simulink model "DP_MotionRAO"  (Simulink 7.4)
settings: Solver=ode4  StartTime=0.0  StopTime=200  FixedStep=0.05  RelTol=1e-3
undefined symbols (not defined in the file): Hoerner, slcm, vessel
libraries: simulink_extras x6, marine_hydro x3, marine_gnc x3, simulink x1
settings Model: Creator=Thor  LastModifiedBy=Thor
settings OptimizationCC: InlineInvariantSignals=on  InitFltsAndDblsToZero=on
settings DebuggingCC: SaveWithParameterizedLinksMsg=none  SignalResolutionControl=TryResolveAllWithWarning  MultiTaskDSMMsg=warning  MultiTaskCondExecSysMsg=none  StrictBusMsg=None
settings RTWCC: IncludeERTFirstTime=on
settings GRTTargetCC: TargetFcnLib=ansi_tfl_tmw.mat

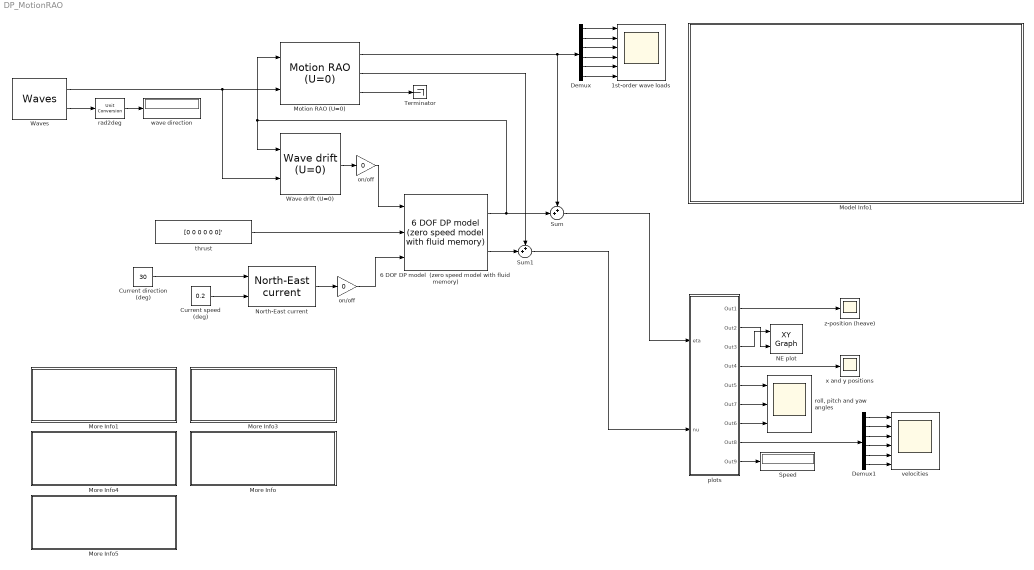
== system DP_MotionRAO ==
  "1st-order wave loads " : Scope  NumInputPorts=6
      settings: TimeRange=200  YMin=-2~-2~-2~-0.4~-0.1~-0.02  YMax=2~1~2~0.4~0.1~0.02
  6 DOF DP model  (zero speed model with fluid memory) : marine_hydro/Hydro Library/6 DOF DP model  (zero speed model with fluid memory)  SystemSampleTime=-1  ABC=vesselABC  rho=1025  Axc=106  Ayc=419  CX=1.0  CY_2D=Hoerner(vessel.main.B,vessel.main.T)  Bv=vessel.Bv
  Current direction (deg) : Constant  Value=30  OutDataType=sfix(16)  OutScaling=2^0
  Current speed (deg) : Constant  Value=0.2  OutDataType=sfix(16)  OutScaling=2^0
  Demux : Demux  Outputs=6
  Demux1 : Demux  Outputs=6
  Model Info1 : Subsystem  LoadFcn=slcm LoadBlock;  InitFcn=slcm('UpdateAllCMBlocksInThisModelInit')  mask(CMBlock){InitialSaveTempField=, InitialBlockCM=None, BlockCM=None, Frame=on, SaveTempField=, DisplayStringWithTags=|, MaskDisplayString=DP_MotionRAO.mdl template (Zero Speed DP Vessel Simulator using MOTION RAOs)\n\nSave this file to your working catalogue before you start editing\n\nVessel simulator for low-speed maneuvering and station-keeping in 6 DOF based on frequency-dependent\nhydrodynamic data. The wave loads and the fluid memory effects are computed using ShipX (VERES) or\nWAMIT that are postprocessed according to:\n\n>>vessel = veres2vessel ('input')        generates the vessel/hydrodynamic data structure <vessel> and *.mat \n>>vessel = wamit2vessel ('myship'')   generates the vessel/hydrodynamic data structure <vessel> and *.mat \n\n>>vesselABC = vessel2ss( vessel )     generates the fluid memory structure <vesselABC> and *ABC.mat\n\nThe data structures <vesselABC> and <vessel> must be in the workspace before starting the simulation\n\nDownload link: www.marinecontrol.org\n\nAuthor: Thor I. Fossen\n17-Sep-2009 10:25:38, HorizontalTextAlignment=Left, LeftAlignmentValue=0.02, SourceBlockDiagram=DP_MotionRAO, TagMaxNumber=20, CMTag1=, CMTag2=, CMTag3=, CMTag4=, CMTag5=, CMTag6=, CMTag7=, CMTag8=, CMTag9=, CMTag10=, CMTag11=, CMTag12=, CMTag13=, CMTag14=, CMTag15=, CMTag16=, CMTag17=, CMTag18=, CMTag19=, CMTag20=}
      mask DisplayStringWithTags=|
      | DP_MotionRAO.mdl template (Zero Speed DP Vessel Simulator using MOTION RAOs)\n
      | Save this file to your working catalogue before you start editing\n
      | Vessel simulator for low-speed maneuvering and station-keeping in 6 DOF based on frequency-dependent\nhydrodynamic data. The wave loads and the fluid memory effects are computed using ShipX (VERES) or\nWAMIT that are postprocessed according to:\n
      | >>vessel = veres2vessel ('input')        generates the vessel/hydrodynamic data structure <vessel> and *.mat
      | >>vessel = wamit2vessel ('myship'')   generates the vessel/hydrodynamic data structure <vessel> and *.mat
      |
      | >>vesselABC = vessel2ss( vessel )     generates the fluid memory structure <vesselABC> and *ABC.mat
      |
      | The data structures <vesselABC> and <vessel> must be in the workspace before starting the simulation
      |
      | Download link: www.marinecontrol.org
      |
      | Author: Thor I. Fossen
      | %<LastModificationDate>
      mask help: This block allows revision control information to be displayed within the model.
      settings: CopyFcn=slcm CopyBlock;  DeleteFcn=slcm Cancel;  PostSaveFcn=slcm('UpdateAllCMBlocksInThisModel')  NameChangeFcn=slcm Rename;  OpenFcn=slcm
      mask Display: text(str2num(LeftAlignmentValue), 0.5, MaskDisplayString, 'HorizontalAlignment', HorizontalTextAlignment)
  More Info : Subsystem
      settings: OpenFcn=load('supply'),load('supplyABC');disp('MSS supply vessel data set (L = 82.80 m) loaded')
      mask Display: disp('ShipX: Supply Vessel (L = 82.80 m)\n  Double-click to load the MSS data files:\n supply.mat\n supplyABC.mat')
  More Info1 : Subsystem
      settings: OpenFcn=load('tanker'),load('tankerABC');disp('MSS tanker data set (L = 246.0 m) loaded')
      mask Display: disp('WAMIT: Tanker (L = 246.0 m)\n  Double-click to load the MSS data files:\n tanker.mat\n tankerABC.mat')
  More Info3 : Subsystem
      settings: OpenFcn=load('s175'),load('s175ABC');disp('MSS S175 data set (L = 175.0 m) loaded')
      mask Display: disp('ShipX: S175 (L = 175.0 m)\n  Double-click to load the MSS data files:\n s175.mat\n s175ABC.mat')
  More Info4 : Subsystem
      settings: OpenFcn=load('fpso'),load('fpsoABC');disp('MSS FPSO data set (L = 200.0 m) loaded')
      mask Display: disp('WAMIT: FPSO (L = 200.0 m)\n  Double-click to load the MSS data files:\n fpso.mat\n fpsoABC.mat')
  More Info5 : Subsystem
      settings: OpenFcn=load('semisub'),load('semisubABC');disp('MSS semi-sub data set (L = 115.0 m) loaded')
      mask Display: disp('WAMIT: Semi-sub (L = 115.0 m)\n  Double-click to load the MSS data files:\n semisub.mat\n semisubABC.mat')
  Motion RAO (U=0) : marine_hydro/Hydro Library/Motion RAO (U=0)  SystemSampleTime=-1  RAO_Freq=vessel.motionRAO.w  RAO_Dir=vessel.headings  RAO_Vel=vessel.velocities  RAO_Amp=vessel.motionRAO.amp  RAO_Phase=vessel.motionRAO.phase  RAO_add_omega_0=on  RAO_add_omega_inf=on  RAO_yaw_quantization_flag=on  RAO_yaw_quant=5*pi/180  RAO_yaw_back=1.2*pi/180  RAO_speed_backlash_flag=on  RAO_speed_back=2  RAO_smoothing_flag=on
  NE plot : simulink/Sinks/XY Graph  SystemSampleTime=-1  xmin=-50  xmax=50  ymin=-50  ymax=50  st=-1
  North-East current : marine_gnc/Environment/Current/North-East current  SystemSampleTime=-1
  Speed : Display
  Sum : Sum  Inputs=++|  OutDataType=sfix(16)  OutScaling=2^0
  Sum1 : Sum  Inputs=++|  OutDataType=sfix(16)  OutScaling=2^0
  Terminator : Terminator
  Wave drift (U=0) : marine_hydro/Hydro Library/Wave drift (U=0)  SystemSampleTime=-1
  Waves : marine_gnc/Environment/Waves/Waves  SystemSampleTime=-1  spectrum_type=ITTC  disp_flag=off  plot_spectrum=off  plot_realization=off  hs=5  omega_peak=-1  psi_mean=30/(180/pi)  gamma=-1  spread=2  depth=inf  nfreq=20  ndir=10  energylim=0.005  freq_cutoff=3  dir_cutoff=0  rand_seed=0  rand_freq=on  rand_dir=on  Zeta_a=0  Omega=0  Phase=0  Wavenum=0  Psi=0
  on/off : Gain  Gain=0  ParameterDataType=sfix(16)  ParameterScaling=2^0  OutDataType=sfix(16)  OutScaling=2^0
  "on/off " : Gain  Gain=0  ParameterDataType=sfix(16)  ParameterScaling=2^0  OutDataType=sfix(16)  OutScaling=2^0
  plots : Subsystem
      mask Display: disp('time-series')
  rad2deg : marine_gnc/Utilities/Math Operations/Unit Conversion  SystemSampleTime=-1  in=rad2deg
  "roll, pitch and yaw angles" : Scope  NumInputPorts=3
      settings: TimeRange=200  YMin=-2~-4~-5  YMax=4~4~10
  thrust : Constant  Value=[0 0 0 0 0 0]'  OutDataType=sfix(16)  OutScaling=2^0
  velocities : Scope  NumInputPorts=6
      settings: TimeRange=200  YMin=-0.5~-0.4~-0.5~-5~-2.5~-1  YMax=0.6~0.5~0.5~5~2.5~1.25  SaveName=ScopeData4
  wave direction : Display
  x and y positions : Scope
      settings: TimeRange=200  YMin=-3  YMax=3  SaveName=ScopeData2
  z-position (heave) : Scope
      settings: TimeRange=200  YMin=-1  YMax=1  SaveName=ScopeData3
  wires:
  thrust/1 -> 6 DOF DP model  (zero speed model with fluid memory)/2
  6 DOF DP model  (zero speed model with fluid memory)/1 -> Sum/2, Motion RAO (U=0)/1, Wave drift (U=0)/1
  Demux/1 -> "1st-order wave loads "/1
  Demux/2 -> "1st-order wave loads "/2
  Demux/3 -> "1st-order wave loads "/3
  Demux/4 -> "1st-order wave loads "/4
  Demux/5 -> "1st-order wave loads "/5
  Demux/6 -> "1st-order wave loads "/6
  Waves/1 -> Motion RAO (U=0)/2, Wave drift (U=0)/2
  Waves/2 -> rad2deg/1
  rad2deg/1 -> wave direction/1
  Motion RAO (U=0)/1 -> Demux/1, Sum/1
  6 DOF DP model  (zero speed model with fluid memory)/2 -> Sum1/2
  Motion RAO (U=0)/2 -> Sum1/1
  Motion RAO (U=0)/3 -> Terminator/1
  North-East current/1 -> "on/off "/1
  "on/off "/1 -> 6 DOF DP model  (zero speed model with fluid memory)/3
  Current speed (deg)/1 -> North-East current/2
  Current direction (deg)/1 -> North-East current/1
  plots/3(Out3) -> NE plot/1
  plots/2(Out2) -> NE plot/2
  plots/4(Out4) -> x and y positions/1
  plots/5(Out5) -> "roll, pitch and yaw angles"/1
  plots/6(Out7) -> "roll, pitch and yaw angles"/2
  plots/7(Out6) -> "roll, pitch and yaw angles"/3
  plots/1(Out1) -> z-position (heave)/1
  Demux1/1 -> velocities/1
  Demux1/2 -> velocities/2
  Demux1/3 -> velocities/3
  Demux1/4 -> velocities/4
  Demux1/5 -> velocities/5
  Demux1/6 -> velocities/6
  Sum1/1 -> plots/2(nu)
  plots/8(Out8) -> Demux1/1
  plots/9(Out9) -> Speed/1
  Sum/1 -> plots/1(eta)
  on/off/1 -> 6 DOF DP model  (zero speed model with fluid memory)/1
  Wave drift (U=0)/1 -> on/off/1

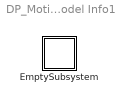
== system DP_MotionRAO/Model Info1 ==
  EmptySubsystem : Subsystem

== system DP_MotionRAO/More Info ==

== system DP_MotionRAO/More Info1 ==

== system DP_MotionRAO/More Info3 ==

== system DP_MotionRAO/More Info4 ==

== system DP_MotionRAO/More Info5 ==

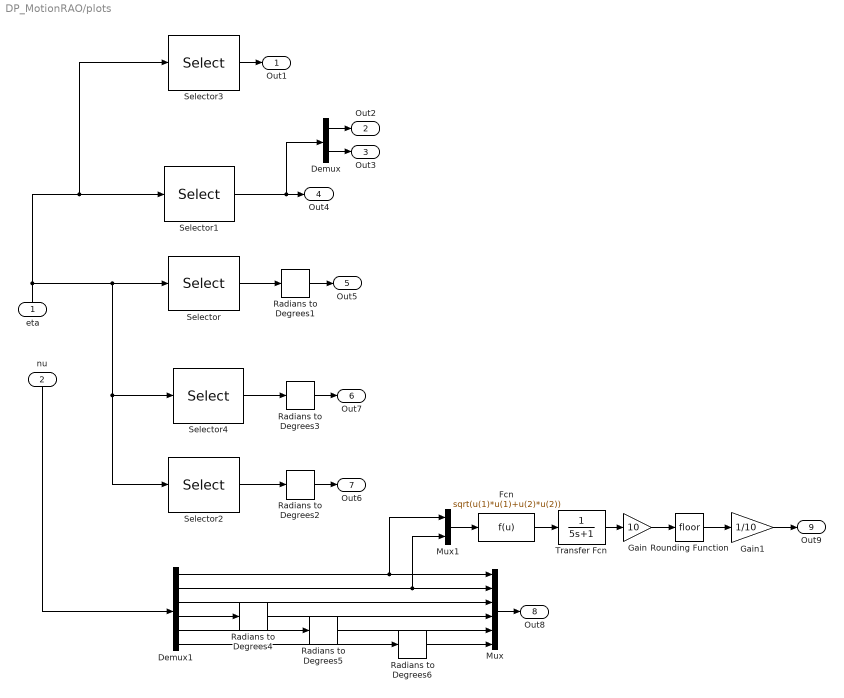
== system DP_MotionRAO/plots ==
  eta : Inport  OutDataType=sfix(16)  OutScaling=2^0
  nu : Inport  Port=2  OutDataType=sfix(16)  OutScaling=2^0
  Demux : Demux  Outputs=2
  Demux1 : Demux  Outputs=6
  Fcn : Fcn  Expr=sqrt(u(1)*u(1)+u(2)*u(2))
  Gain : Gain  Gain=10  ParameterDataType=sfix(16)  ParameterScaling=2^0  OutDataType=sfix(16)  OutScaling=2^0
  Gain1 : Gain  Gain=1/10  ParameterDataType=sfix(16)  ParameterScaling=2^0  OutDataType=sfix(16)  OutScaling=2^0
  Mux : Mux  Inputs=6
  Mux1 : Mux  Inputs=2
  Radians to Degrees{1..6} (6 alike) : simulink_extras/Transformations/Radians to Degrees  SystemSampleTime=-1
  Rounding Function : Rounding
  Selector : Selector  InputPortWidth=6  IndexOptions=Index vector (dialog)  Indices=[4 ]  OutputSizes=1
  Selector1 : Selector  InputPortWidth=6  IndexOptions=Index vector (dialog)  Indices=[1 2]  OutputSizes=1
  Selector2 : Selector  InputPortWidth=6  IndexOptions=Index vector (dialog)  Indices=[6]  OutputSizes=1
  Selector3 : Selector  InputPortWidth=6  IndexOptions=Index vector (dialog)  Indices=[3]  OutputSizes=1
  Selector4 : Selector  InputPortWidth=6  IndexOptions=Index vector (dialog)  Indices=[5]  OutputSizes=1
  Transfer Fcn : TransferFcn  Denominator=[5 1]
  Out1 : Outport  OutDataType=sfix(16)  OutScaling=2^0
  Out2 : Outport  Port=2  OutDataType=sfix(16)  OutScaling=2^0
  Out3 : Outport  Port=3  OutDataType=sfix(16)  OutScaling=2^0
  Out4 : Outport  Port=4  OutDataType=sfix(16)  OutScaling=2^0
  Out5 : Outport  Port=5  OutDataType=sfix(16)  OutScaling=2^0
  Out7 : Outport  Port=6  OutDataType=sfix(16)  OutScaling=2^0
  Out6 : Outport  Port=7  OutDataType=sfix(16)  OutScaling=2^0
  Out8 : Outport  Port=8  OutDataType=sfix(16)  OutScaling=2^0
  Out9 : Outport  Port=9  OutDataType=sfix(16)  OutScaling=2^0
  wires:
  eta/1 -> Selector3/1, Selector1/1, Selector/1, Selector2/1, Selector4/1
  Selector/1 -> Radians to Degrees1/1
  Selector1/1 -> Demux/1, Out4/1
  Selector2/1 -> Radians to Degrees2/1
  Selector3/1 -> Out1/1
  Demux/1 -> Out2/1
  Demux/2 -> Out3/1
  Radians to Degrees1/1 -> Out5/1
  Radians to Degrees2/1 -> Out6/1
  Selector4/1 -> Radians to Degrees3/1
  Radians to Degrees3/1 -> Out7/1
  nu/1 -> Demux1/1
  Demux1/1 -> Mux/1, Mux1/1
  Demux1/2 -> Mux/2, Mux1/2
  Demux1/3 -> Mux/3
  Demux1/4 -> Radians to Degrees4/1
  Demux1/5 -> Radians to Degrees5/1
  Demux1/6 -> Radians to Degrees6/1
  Radians to Degrees6/1 -> Mux/6
  Radians to Degrees5/1 -> Mux/5
  Radians to Degrees4/1 -> Mux/4
  Mux/1 -> Out8/1
  Fcn/1 -> Transfer Fcn/1
  Mux1/1 -> Fcn/1
  Rounding Function/1 -> Gain1/1
  Gain/1 -> Rounding Function/1
  Gain1/1 -> Out9/1
  Transfer Fcn/1 -> Gain/1

== system DP_MotionRAO/Model Info1/EmptySubsystem ==
